simulink model "multicoptero"  (R2024b)
settings: Solver=FixedStepAuto  StartTime=0.0  StopTime=10  FixedStep=1e-3  RelTol=1e-3
undefined symbols (not defined in the file or in its folder): carga, controlador, planta
libraries: slpidlib x6
settings Model: Creator=mmaximo  LastModifiedBy=guicr
settings SolverCC: AlgebraicLoopSolver=TrustRegion
settings DebuggingCC: UnconnectedInputMsg=warning  UnconnectedOutputMsg=warning  UnconnectedLineMsg=warning
settings ModelReferenceCC: EnableRefExpFcnMdlSchedulingChecks=on
settings RTWCC: GPUComputeCapability=3.5

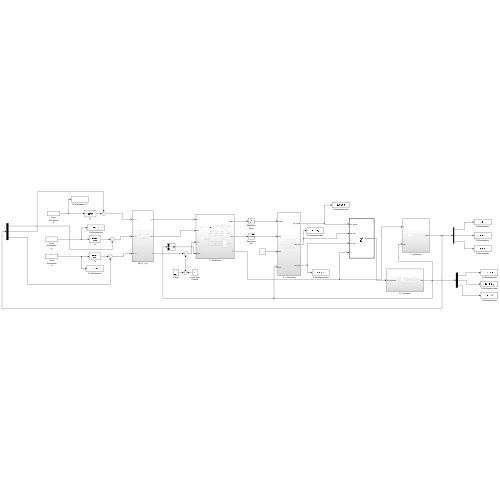
[thumbnail: Simulink's stored preview of the top-level diagram]
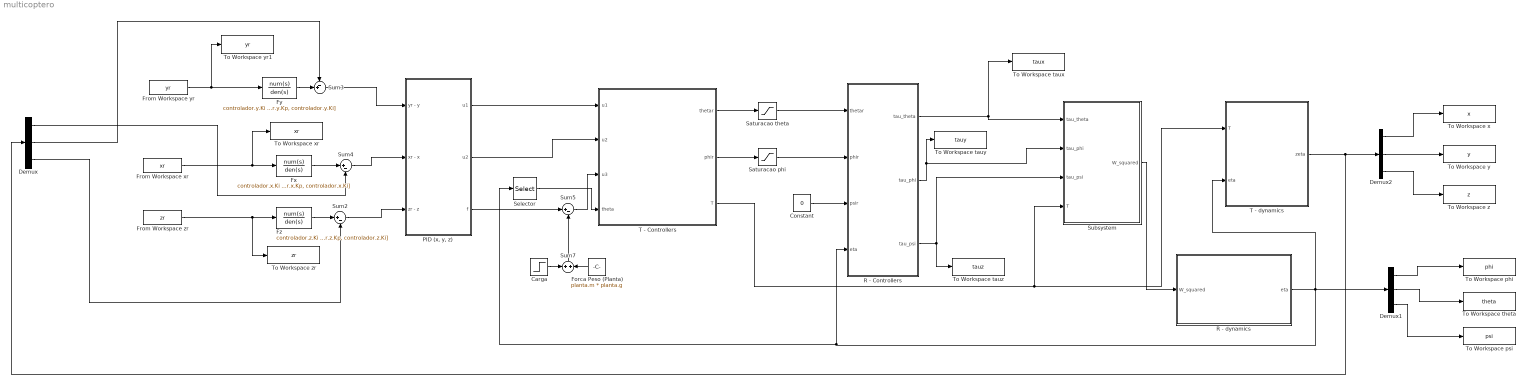
== system multicoptero ==
  Carga : Step  Time=3  After=carga * planta.g  SampleTime=0
  Constant : Constant  Value=0
  Demux : Demux  Outputs=3
  Demux1 : Demux  Outputs=3
  Demux2 : Demux  Outputs=3
  Forca Peso (Planta) : Constant  Value=planta.m * planta.g
  From Workspace xr : FromWorkspace  VariableName=xr
  From Workspace yr : FromWorkspace  VariableName=yr
  From Workspace zr : FromWorkspace  VariableName=zr
  Fx : TransferFcn  Numerator=controlador.x.Ki  Denominator=[controlador.x.Kd, controlador.x.Kp, controlador.x.Ki]
  Fy : TransferFcn  Numerator=controlador.y.Ki  Denominator=[controlador.y.Kd, controlador.y.Kp, controlador.y.Ki]
  Fz : TransferFcn  Numerator=controlador.z.Ki  Denominator=[controlador.z.Kd, controlador.z.Kp, controlador.z.Ki]
  "PID (x, y, z)" : Subsystem
  R - Controllers : Subsystem
  R - dynamics : Subsystem
  Saturacao phi : Saturate  UpperLimit=80 * pi / 180  LowerLimit=-80 * pi / 180
  Saturacao theta : Saturate  UpperLimit=80 * pi / 180  LowerLimit=-80 * pi / 180
  Selector : Selector  InputPortWidth=3  IndexOptions=Index vector (dialog)  Indices=[2]  OutputSizes=1
  Subsystem : MATLAB Function  TreatAsAtomicUnit=on
  Sum2 : Sum  Inputs=|+-
  Sum3 : Sum  Inputs=-+|
  Sum4 : Sum  Inputs=|+-
  Sum5 : Sum  Inputs=|+-
  Sum7 : Sum  Inputs=+|+
  T - Controllers : Subsystem
  T - dynamics : Subsystem
  To Workspace phi : ToWorkspace  VariableName=phi  SaveFormat=Structure With Time  SampleTime=-1
  To Workspace psi : ToWorkspace  VariableName=psi  SaveFormat=Structure With Time  SampleTime=-1
  To Workspace taux : ToWorkspace  VariableName=taux  SaveFormat=Structure With Time  SampleTime=-1
  To Workspace tauy : ToWorkspace  VariableName=tauy  SaveFormat=Structure With Time  SampleTime=-1
  To Workspace tauz : ToWorkspace  VariableName=tauz  SaveFormat=Structure With Time  SampleTime=-1
  To Workspace theta : ToWorkspace  VariableName=theta  SaveFormat=Structure With Time  SampleTime=-1
  To Workspace x : ToWorkspace  VariableName=x  SaveFormat=Structure With Time  SampleTime=-1
  To Workspace xr : ToWorkspace  VariableName=xr  SaveFormat=Structure With Time  SampleTime=-1
  To Workspace y : ToWorkspace  VariableName=y  SaveFormat=Structure With Time  SampleTime=-1
  To Workspace yr1 : ToWorkspace  VariableName=yr  SaveFormat=Structure With Time  SampleTime=-1
  To Workspace z : ToWorkspace  VariableName=z  SaveFormat=Structure With Time  SampleTime=-1
  To Workspace zr : ToWorkspace  VariableName=zr  SaveFormat=Structure With Time  SampleTime=-1
  wires:
  From Workspace yr/1 -> To Workspace yr1/1, Fy/1
  From Workspace zr/1 -> Fz/1, To Workspace zr/1
  Fz/1 -> Sum2/1
  Fx/1 -> Sum4/1
  From Workspace xr/1 -> To Workspace xr/1, Fx/1
  Fy/1 -> Sum3/2
  Sum3/1 -> "PID (x, y, z)"/1(yr - y)
  Sum4/1 -> "PID (x, y, z)"/2(xr - x)
  Sum2/1 -> "PID (x, y, z)"/3(zr - z)
  Forca Peso (Planta)/1 -> Sum7/2
  Sum7/1 -> Sum5/2
  Carga/1 -> Sum7/1
  "PID (x, y, z)"/3(f) -> Sum5/1
  "PID (x, y, z)"/1(u1) -> T - Controllers/1(u1)
  "PID (x, y, z)"/2(u2) -> T - Controllers/2(u2)
  Sum5/1 -> T - Controllers/3(u3)
  T - Controllers/1(thetar) -> Saturacao theta/1
  T - Controllers/2(phir) -> Saturacao phi/1
  Constant/1 -> R - Controllers/3(psir)
  R - Controllers/2(tau_phi) -> Subsystem/2(tau_phi), To Workspace tauy/1
  R - Controllers/1(tau_theta) -> To Workspace taux/1, Subsystem/1(tau_theta)
  R - Controllers/3(tau_psi) -> To Workspace tauz/1, Subsystem/3(tau_psi)
  Subsystem/1(W_squared) -> R - dynamics/1(W_squared)
  Demux/3 -> Sum2/2
  Demux/1 -> Sum4/2
  Demux/2 -> Sum3/1
  R - dynamics/1(eta) -> Selector/1, R - Controllers/4(eta), Demux1/1, T - dynamics/2(eta)
  T - dynamics/1(zeta) -> Demux/1, Demux2/1
  Saturacao theta/1 -> R - Controllers/1(thetar)
  Saturacao phi/1 -> R - Controllers/2(phir)
  Demux1/1 -> To Workspace phi/1
  Demux1/2 -> To Workspace theta/1
  Demux1/3 -> To Workspace psi/1
  Demux2/1 -> To Workspace x/1
  Demux2/2 -> To Workspace y/1
  Demux2/3 -> To Workspace z/1
  T - Controllers/3(T) -> T - dynamics/1(T), Subsystem/4(T)
  Selector/1 -> T - Controllers/4(theta)

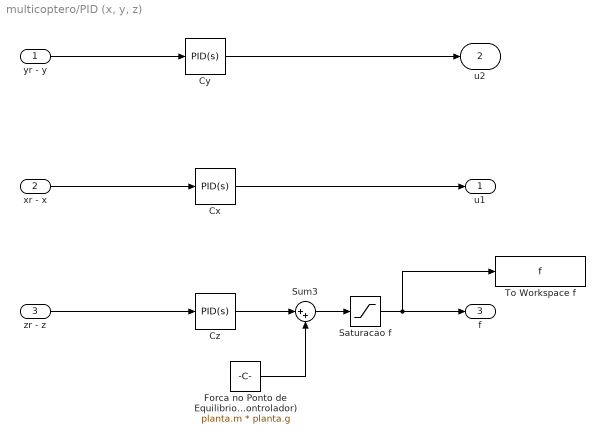
== system multicoptero/PID (x, y, z) ==
  yr - y : Inport
  xr - x : Inport  Port=2
  zr - z : Inport  Port=3
  Cx : slpidlib/PID Controller  Controller=PID  Form=Parallel  TimeDomain=Continuous-time  UseExternalTs=off  SampleTime=-1  IntegratorMethod=Forward Euler  FilterMethod=Forward Euler  ControllerParametersSource=internal  P=controlador.x.Kp  I=controlador.x.Ki  UseKiTs=off  D=controlador.x.Kd  UseExternalDerivativeSource=off  N=100  UseFilter=on  TunerSelectOption=Transfer Function Based (PID Tuner App)  InitialConditionSource=internal  InitialConditionForIntegrator=0  InitialConditionForFilter=0  DifferentiatorICPrevScaledInput=0  ExternalReset=none  TrackingMode=off  Kt=1  LimitOutput=off  SatLimitsSource=internal  UpperSaturationLimit=inf  LowerSaturationLimit=-inf  LinearizeAsGain=on  AntiWindupMode=none  Kb=1  LimitIntegrator=off  UpperIntegratorSaturationLimit=inf  LowerIntegratorSaturationLimit=-inf  POutMin=[]  POutMax=[]  IOutMin=[]  IOutMax=[]  DOutMin=[]  DOutMax=[]  NOutMin=[]  NOutMax=[]  SumOutMin=[]  SumOutMax=[]  SaturationOutMin=[]  SaturationOutMax=[]  PParamMin=[]  PParamMax=[]  IParamMin=[]  IParamMax=[]  DParamMin=[]  DParamMax=[]  NParamMin=[]  NParamMax=[]  KbParamMin=[]  KbParamMax=[]  KtParamMin=[]  KtParamMax=[]  KbOutMin=[]  KbOutMax=[]  KtOutMin=[]  KtOutMax=[]  IntegratorOutMin=[]  IntegratorOutMax=[]  FilterOutMin=[]  FilterOutMax=[]  SumI1OutMin=[]  SumI1OutMax=[]  SumI2OutMin=[]  SumI2OutMax=[]  SumI3OutMin=[]  SumI3OutMax=[]  SumI4OutMin=[]  SumI4OutMax=[]  SumDOutMin=[]  SumDOutMax=[]  DifferentiatorOutMin=[]  DifferentiatorOutMax=[]  FilterDiffOutCoefMin=[]  FilterDiffOutCoefMax=[]  ReciprocalOutMin=[]  ReciprocalOutMax=[]  SumDenOutMin=[]  SumDenOutMax=[]  SumNumOutMin=[]  SumNumOutMax=[]  DivideOutMin=[]  DivideOutMax=[]  UdiffTsProdOutMin=[]  UdiffTsProdOutMax=[]  NTsProdOutMin=[]  NTsProdOutMax=[]  UintegralTsProdOutMin=[]  UintegralTsProdOutMax=[]  UngainTsProdOutMin=[]  UngainTsProdOutMax=[]  ClampingZeroOutDataTypeStr=Inherit: Inherit via back propagation  ClampingZeroOutMin=[]  ClampingZeroOutMax=[]  FilterDenConstantOutDataTypeStr=Inherit: Inherit via back propagation  FilterDenConstantOutMin=[]  FilterDenConstantOutMax=[]  PCopyOutDataTypeStr=Inherit: Inherit via back propagation  PCopyOutMin=[]  PCopyOutMax=[]  NCopyOutDataTypeStr=Inherit: Inherit via back propagation  NCopyOutMin=[]  NCopyOutMax=[]  IntegratorContinuousStateAttributes=''  IntegratorStateMustResolveToSignalObject=off  IntegratorRTWStateStorageClass=Auto  FilterContinuousStateAttributes=''  FilterStateMustResolveToSignalObject=off  FilterRTWStateStorageClass=Auto  ParallelPVariant=InternalParameters  IdealPVariant=Disabled  IVariant=InternalParameters  DVariant=InternalParameters  IntegratorVariant=Continuous  SatVariant=Disabled  AWVariant=Passthrough  PCopyVariant=Disabled  TRVariant=Disabled  FdbkBlocksVariant=Forward  IdealPFdbkVariant=Disabled  SatFdbkVariant=Disabled  DerivativeFilterVariant=ContFilter  NVariant=InternalParameters  NCopyVariant=Disabled  FilterICVariant=InternalICsFilter  IntegratorICVariant=InternalICs  ExternalResetVariant=Disabled  TRSumVariant=Passthrough  SumFdbkVariant=Disabled  SumVariant=Sum_PID  TsampFilterVariant=InternalTs  TsampNgainVariant=Passthrough  TsampIntegralVariant=Disabled_SignalSpec  ExternalSaturationOutDataTypeStr=Inherit: Same as second input  DerivativeSourceVariant=ErrorSignal  PreIntVariant=InternalPreInt
  Cy : slpidlib/PID Controller  Controller=PID  Form=Parallel  TimeDomain=Continuous-time  UseExternalTs=off  SampleTime=-1  IntegratorMethod=Forward Euler  FilterMethod=Forward Euler  ControllerParametersSource=internal  P=controlador.y.Kp  I=controlador.y.Ki  UseKiTs=off  D=controlador.y.Kd  UseExternalDerivativeSource=off  N=100  UseFilter=on  TunerSelectOption=Transfer Function Based (PID Tuner App)  InitialConditionSource=internal  InitialConditionForIntegrator=0  InitialConditionForFilter=0  DifferentiatorICPrevScaledInput=0  ExternalReset=none  TrackingMode=off  Kt=1  LimitOutput=off  SatLimitsSource=internal  UpperSaturationLimit=inf  LowerSaturationLimit=-inf  LinearizeAsGain=on  AntiWindupMode=none  Kb=1  LimitIntegrator=off  UpperIntegratorSaturationLimit=inf  LowerIntegratorSaturationLimit=-inf  POutMin=[]  POutMax=[]  IOutMin=[]  IOutMax=[]  DOutMin=[]  DOutMax=[]  NOutMin=[]  NOutMax=[]  SumOutMin=[]  SumOutMax=[]  SaturationOutMin=[]  SaturationOutMax=[]  PParamMin=[]  PParamMax=[]  IParamMin=[]  IParamMax=[]  DParamMin=[]  DParamMax=[]  NParamMin=[]  NParamMax=[]  KbParamMin=[]  KbParamMax=[]  KtParamMin=[]  KtParamMax=[]  KbOutMin=[]  KbOutMax=[]  KtOutMin=[]  KtOutMax=[]  IntegratorOutMin=[]  IntegratorOutMax=[]  FilterOutMin=[]  FilterOutMax=[]  SumI1OutMin=[]  SumI1OutMax=[]  SumI2OutMin=[]  SumI2OutMax=[]  SumI3OutMin=[]  SumI3OutMax=[]  SumI4OutMin=[]  SumI4OutMax=[]  SumDOutMin=[]  SumDOutMax=[]  DifferentiatorOutMin=[]  DifferentiatorOutMax=[]  FilterDiffOutCoefMin=[]  FilterDiffOutCoefMax=[]  ReciprocalOutMin=[]  ReciprocalOutMax=[]  SumDenOutMin=[]  SumDenOutMax=[]  SumNumOutMin=[]  SumNumOutMax=[]  DivideOutMin=[]  DivideOutMax=[]  UdiffTsProdOutMin=[]  UdiffTsProdOutMax=[]  NTsProdOutMin=[]  NTsProdOutMax=[]  UintegralTsProdOutMin=[]  UintegralTsProdOutMax=[]  UngainTsProdOutMin=[]  UngainTsProdOutMax=[]  ClampingZeroOutDataTypeStr=Inherit: Inherit via back propagation  ClampingZeroOutMin=[]  ClampingZeroOutMax=[]  FilterDenConstantOutDataTypeStr=Inherit: Inherit via back propagation  FilterDenConstantOutMin=[]  FilterDenConstantOutMax=[]  PCopyOutDataTypeStr=Inherit: Inherit via back propagation  PCopyOutMin=[]  PCopyOutMax=[]  NCopyOutDataTypeStr=Inherit: Inherit via back propagation  NCopyOutMin=[]  NCopyOutMax=[]  IntegratorContinuousStateAttributes=''  IntegratorStateMustResolveToSignalObject=off  IntegratorRTWStateStorageClass=Auto  FilterContinuousStateAttributes=''  FilterStateMustResolveToSignalObject=off  FilterRTWStateStorageClass=Auto  ParallelPVariant=InternalParameters  IdealPVariant=Disabled  IVariant=InternalParameters  DVariant=InternalParameters  IntegratorVariant=Continuous  SatVariant=Disabled  AWVariant=Passthrough  PCopyVariant=Disabled  TRVariant=Disabled  FdbkBlocksVariant=Forward  IdealPFdbkVariant=Disabled  SatFdbkVariant=Disabled  DerivativeFilterVariant=ContFilter  NVariant=InternalParameters  NCopyVariant=Disabled  FilterICVariant=InternalICsFilter  IntegratorICVariant=InternalICs  ExternalResetVariant=Disabled  TRSumVariant=Passthrough  SumFdbkVariant=Disabled  SumVariant=Sum_PID  TsampFilterVariant=InternalTs  TsampNgainVariant=Passthrough  TsampIntegralVariant=Disabled_SignalSpec  ExternalSaturationOutDataTypeStr=Inherit: Same as second input  DerivativeSourceVariant=ErrorSignal  PreIntVariant=InternalPreInt
  Cz : slpidlib/PID Controller  Controller=PID  Form=Parallel  TimeDomain=Continuous-time  UseExternalTs=off  SampleTime=-1  IntegratorMethod=Forward Euler  FilterMethod=Forward Euler  ControllerParametersSource=internal  P=controlador.z.Kp  I=controlador.z.Ki  UseKiTs=off  D=controlador.z.Kd  UseExternalDerivativeSource=off  N=100  UseFilter=on  TunerSelectOption=Transfer Function Based (PID Tuner App)  InitialConditionSource=internal  InitialConditionForIntegrator=0  InitialConditionForFilter=0  DifferentiatorICPrevScaledInput=0  ExternalReset=none  TrackingMode=off  Kt=1  LimitOutput=off  SatLimitsSource=internal  UpperSaturationLimit=inf  LowerSaturationLimit=-inf  LinearizeAsGain=on  AntiWindupMode=none  Kb=1  LimitIntegrator=off  UpperIntegratorSaturationLimit=inf  LowerIntegratorSaturationLimit=-inf  POutMin=[]  POutMax=[]  IOutMin=[]  IOutMax=[]  DOutMin=[]  DOutMax=[]  NOutMin=[]  NOutMax=[]  SumOutMin=[]  SumOutMax=[]  SaturationOutMin=[]  SaturationOutMax=[]  PParamMin=[]  PParamMax=[]  IParamMin=[]  IParamMax=[]  DParamMin=[]  DParamMax=[]  NParamMin=[]  NParamMax=[]  KbParamMin=[]  KbParamMax=[]  KtParamMin=[]  KtParamMax=[]  KbOutMin=[]  KbOutMax=[]  KtOutMin=[]  KtOutMax=[]  IntegratorOutMin=[]  IntegratorOutMax=[]  FilterOutMin=[]  FilterOutMax=[]  SumI1OutMin=[]  SumI1OutMax=[]  SumI2OutMin=[]  SumI2OutMax=[]  SumI3OutMin=[]  SumI3OutMax=[]  SumI4OutMin=[]  SumI4OutMax=[]  SumDOutMin=[]  SumDOutMax=[]  DifferentiatorOutMin=[]  DifferentiatorOutMax=[]  FilterDiffOutCoefMin=[]  FilterDiffOutCoefMax=[]  ReciprocalOutMin=[]  ReciprocalOutMax=[]  SumDenOutMin=[]  SumDenOutMax=[]  SumNumOutMin=[]  SumNumOutMax=[]  DivideOutMin=[]  DivideOutMax=[]  UdiffTsProdOutMin=[]  UdiffTsProdOutMax=[]  NTsProdOutMin=[]  NTsProdOutMax=[]  UintegralTsProdOutMin=[]  UintegralTsProdOutMax=[]  UngainTsProdOutMin=[]  UngainTsProdOutMax=[]  ClampingZeroOutDataTypeStr=Inherit: Inherit via back propagation  ClampingZeroOutMin=[]  ClampingZeroOutMax=[]  FilterDenConstantOutDataTypeStr=Inherit: Inherit via back propagation  FilterDenConstantOutMin=[]  FilterDenConstantOutMax=[]  PCopyOutDataTypeStr=Inherit: Inherit via back propagation  PCopyOutMin=[]  PCopyOutMax=[]  NCopyOutDataTypeStr=Inherit: Inherit via back propagation  NCopyOutMin=[]  NCopyOutMax=[]  IntegratorContinuousStateAttributes=''  IntegratorStateMustResolveToSignalObject=off  IntegratorRTWStateStorageClass=Auto  FilterContinuousStateAttributes=''  FilterStateMustResolveToSignalObject=off  FilterRTWStateStorageClass=Auto  ParallelPVariant=InternalParameters  IdealPVariant=Disabled  IVariant=InternalParameters  DVariant=InternalParameters  IntegratorVariant=Continuous  SatVariant=Disabled  AWVariant=Passthrough  PCopyVariant=Disabled  TRVariant=Disabled  FdbkBlocksVariant=Forward  IdealPFdbkVariant=Disabled  SatFdbkVariant=Disabled  DerivativeFilterVariant=ContFilter  NVariant=InternalParameters  NCopyVariant=Disabled  FilterICVariant=InternalICsFilter  IntegratorICVariant=InternalICs  ExternalResetVariant=Disabled  TRSumVariant=Passthrough  SumFdbkVariant=Disabled  SumVariant=Sum_PID  TsampFilterVariant=InternalTs  TsampNgainVariant=Passthrough  TsampIntegralVariant=Disabled_SignalSpec  ExternalSaturationOutDataTypeStr=Inherit: Same as second input  DerivativeSourceVariant=ErrorSignal  PreIntVariant=InternalPreInt
  Forca no Ponto de Equilibrio f0 (Controlador) : Constant  Value=planta.m * planta.g
  Saturacao f : Saturate  UpperLimit=1.8 * planta.m * planta.g  LowerLimit=0.2 * planta.m * planta.g
  Sum3 : Sum  Inputs=|++
  To Workspace f : ToWorkspace  VariableName=f  SaveFormat=Structure With Time  SampleTime=-1
  u1 : Outport
  u2 : Outport  Port=2
  f : Outport  Port=3
  wires:
  Forca no Ponto de Equilibrio f0 (Controlador)/1 -> Sum3/2
  Cx/1 -> u1/1
  xr - x/1 -> Cx/1
  Saturacao f/1 -> To Workspace f/1, f/1
  Cz/1 -> Sum3/1
  Cy/1 -> u2/1
  Sum3/1 -> Saturacao f/1
  yr - y/1 -> Cy/1
  zr - z/1 -> Cz/1

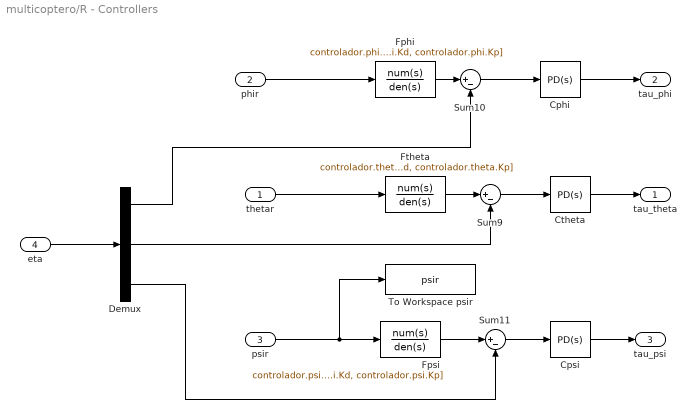
== system multicoptero/R - Controllers ==
  thetar : Inport
  phir : Inport  Port=2
  psir : Inport  Port=3
  eta : Inport  Port=4
  Cphi : slpidlib/PID Controller  Controller=PD  Form=Parallel  TimeDomain=Continuous-time  UseExternalTs=off  SampleTime=-1  IntegratorMethod=Forward Euler  FilterMethod=Forward Euler  ControllerParametersSource=internal  P=controlador.phi.Kp  I=controlador.phi.Ki  UseKiTs=off  D=controlador.phi.Kd  UseExternalDerivativeSource=off  N=100  UseFilter=on  TunerSelectOption=Transfer Function Based (PID Tuner App)  InitialConditionSource=internal  InitialConditionForIntegrator=0  InitialConditionForFilter=0  DifferentiatorICPrevScaledInput=0  ExternalReset=none  TrackingMode=off  Kt=1  LimitOutput=off  SatLimitsSource=internal  UpperSaturationLimit=inf  LowerSaturationLimit=-inf  LinearizeAsGain=on  AntiWindupMode=none  Kb=1  LimitIntegrator=off  UpperIntegratorSaturationLimit=inf  LowerIntegratorSaturationLimit=-inf  POutMin=[]  POutMax=[]  IOutMin=[]  IOutMax=[]  DOutMin=[]  DOutMax=[]  NOutMin=[]  NOutMax=[]  SumOutMin=[]  SumOutMax=[]  SaturationOutMin=[]  SaturationOutMax=[]  PParamMin=[]  PParamMax=[]  IParamMin=[]  IParamMax=[]  DParamMin=[]  DParamMax=[]  NParamMin=[]  NParamMax=[]  KbParamMin=[]  KbParamMax=[]  KtParamMin=[]  KtParamMax=[]  KbOutMin=[]  KbOutMax=[]  KtOutMin=[]  KtOutMax=[]  IntegratorOutMin=[]  IntegratorOutMax=[]  FilterOutMin=[]  FilterOutMax=[]  SumI1OutMin=[]  SumI1OutMax=[]  SumI2OutMin=[]  SumI2OutMax=[]  SumI3OutMin=[]  SumI3OutMax=[]  SumI4OutMin=[]  SumI4OutMax=[]  SumDOutMin=[]  SumDOutMax=[]  DifferentiatorOutMin=[]  DifferentiatorOutMax=[]  FilterDiffOutCoefMin=[]  FilterDiffOutCoefMax=[]  ReciprocalOutMin=[]  ReciprocalOutMax=[]  SumDenOutMin=[]  SumDenOutMax=[]  SumNumOutMin=[]  SumNumOutMax=[]  DivideOutMin=[]  DivideOutMax=[]  UdiffTsProdOutMin=[]  UdiffTsProdOutMax=[]  NTsProdOutMin=[]  NTsProdOutMax=[]  UintegralTsProdOutMin=[]  UintegralTsProdOutMax=[]  UngainTsProdOutMin=[]  UngainTsProdOutMax=[]  ClampingZeroOutDataTypeStr=Inherit: Inherit via back propagation  ClampingZeroOutMin=[]  ClampingZeroOutMax=[]  FilterDenConstantOutDataTypeStr=Inherit: Inherit via back propagation  FilterDenConstantOutMin=[]  FilterDenConstantOutMax=[]  PCopyOutDataTypeStr=Inherit: Inherit via back propagation  PCopyOutMin=[]  PCopyOutMax=[]  NCopyOutDataTypeStr=Inherit: Inherit via back propagation  NCopyOutMin=[]  NCopyOutMax=[]  IntegratorContinuousStateAttributes=''  IntegratorStateMustResolveToSignalObject=off  IntegratorRTWStateStorageClass=Auto  FilterContinuousStateAttributes=''  FilterStateMustResolveToSignalObject=off  FilterRTWStateStorageClass=Auto  ParallelPVariant=InternalParameters  IdealPVariant=Disabled  IVariant=Disabled  DVariant=InternalParameters  IntegratorVariant=Disabled  SatVariant=Disabled  AWVariant=Disabled  PCopyVariant=Disabled  TRVariant=Disabled  FdbkBlocksVariant=Forward  IdealPFdbkVariant=Disabled  SatFdbkVariant=Disabled  DerivativeFilterVariant=ContFilter  NVariant=InternalParameters  NCopyVariant=Disabled  FilterICVariant=InternalICsFilter  IntegratorICVariant=Disabled  ExternalResetVariant=Disabled  TRSumVariant=Passthrough  SumFdbkVariant=Disabled  SumVariant=Sum_PD  TsampFilterVariant=InternalTs  TsampNgainVariant=Passthrough  TsampIntegralVariant=Disabled_SignalSpec  ExternalSaturationOutDataTypeStr=Inherit: Same as second input  DerivativeSourceVariant=ErrorSignal  PreIntVariant=InternalPreInt
  Cpsi : slpidlib/PID Controller  Controller=PD  Form=Parallel  TimeDomain=Continuous-time  UseExternalTs=off  SampleTime=-1  IntegratorMethod=Forward Euler  FilterMethod=Forward Euler  ControllerParametersSource=internal  P=controlador.psi.Kp  I=controlador.psi.Ki  UseKiTs=off  D=controlador.psi.Kd  UseExternalDerivativeSource=off  N=100  UseFilter=on  TunerSelectOption=Transfer Function Based (PID Tuner App)  InitialConditionSource=internal  InitialConditionForIntegrator=0  InitialConditionForFilter=0  DifferentiatorICPrevScaledInput=0  ExternalReset=none  TrackingMode=off  Kt=1  LimitOutput=off  SatLimitsSource=internal  UpperSaturationLimit=inf  LowerSaturationLimit=-inf  LinearizeAsGain=on  AntiWindupMode=none  Kb=1  LimitIntegrator=off  UpperIntegratorSaturationLimit=inf  LowerIntegratorSaturationLimit=-inf  POutMin=[]  POutMax=[]  IOutMin=[]  IOutMax=[]  DOutMin=[]  DOutMax=[]  NOutMin=[]  NOutMax=[]  SumOutMin=[]  SumOutMax=[]  SaturationOutMin=[]  SaturationOutMax=[]  PParamMin=[]  PParamMax=[]  IParamMin=[]  IParamMax=[]  DParamMin=[]  DParamMax=[]  NParamMin=[]  NParamMax=[]  KbParamMin=[]  KbParamMax=[]  KtParamMin=[]  KtParamMax=[]  KbOutMin=[]  KbOutMax=[]  KtOutMin=[]  KtOutMax=[]  IntegratorOutMin=[]  IntegratorOutMax=[]  FilterOutMin=[]  FilterOutMax=[]  SumI1OutMin=[]  SumI1OutMax=[]  SumI2OutMin=[]  SumI2OutMax=[]  SumI3OutMin=[]  SumI3OutMax=[]  SumI4OutMin=[]  SumI4OutMax=[]  SumDOutMin=[]  SumDOutMax=[]  DifferentiatorOutMin=[]  DifferentiatorOutMax=[]  FilterDiffOutCoefMin=[]  FilterDiffOutCoefMax=[]  ReciprocalOutMin=[]  ReciprocalOutMax=[]  SumDenOutMin=[]  SumDenOutMax=[]  SumNumOutMin=[]  SumNumOutMax=[]  DivideOutMin=[]  DivideOutMax=[]  UdiffTsProdOutMin=[]  UdiffTsProdOutMax=[]  NTsProdOutMin=[]  NTsProdOutMax=[]  UintegralTsProdOutMin=[]  UintegralTsProdOutMax=[]  UngainTsProdOutMin=[]  UngainTsProdOutMax=[]  ClampingZeroOutDataTypeStr=Inherit: Inherit via back propagation  ClampingZeroOutMin=[]  ClampingZeroOutMax=[]  FilterDenConstantOutDataTypeStr=Inherit: Inherit via back propagation  FilterDenConstantOutMin=[]  FilterDenConstantOutMax=[]  PCopyOutDataTypeStr=Inherit: Inherit via back propagation  PCopyOutMin=[]  PCopyOutMax=[]  NCopyOutDataTypeStr=Inherit: Inherit via back propagation  NCopyOutMin=[]  NCopyOutMax=[]  IntegratorContinuousStateAttributes=''  IntegratorStateMustResolveToSignalObject=off  IntegratorRTWStateStorageClass=Auto  FilterContinuousStateAttributes=''  FilterStateMustResolveToSignalObject=off  FilterRTWStateStorageClass=Auto  ParallelPVariant=InternalParameters  IdealPVariant=Disabled  IVariant=Disabled  DVariant=InternalParameters  IntegratorVariant=Disabled  SatVariant=Disabled  AWVariant=Disabled  PCopyVariant=Disabled  TRVariant=Disabled  FdbkBlocksVariant=Forward  IdealPFdbkVariant=Disabled  SatFdbkVariant=Disabled  DerivativeFilterVariant=ContFilter  NVariant=InternalParameters  NCopyVariant=Disabled  FilterICVariant=InternalICsFilter  IntegratorICVariant=Disabled  ExternalResetVariant=Disabled  TRSumVariant=Passthrough  SumFdbkVariant=Disabled  SumVariant=Sum_PD  TsampFilterVariant=InternalTs  TsampNgainVariant=Passthrough  TsampIntegralVariant=Disabled_SignalSpec  ExternalSaturationOutDataTypeStr=Inherit: Same as second input  DerivativeSourceVariant=ErrorSignal  PreIntVariant=InternalPreInt
  Ctheta : slpidlib/PID Controller  Controller=PD  Form=Parallel  TimeDomain=Continuous-time  UseExternalTs=off  SampleTime=-1  IntegratorMethod=Forward Euler  FilterMethod=Forward Euler  ControllerParametersSource=internal  P=controlador.theta.Kp  I=controlador.theta.Ki  UseKiTs=off  D=controlador.theta.Kd  UseExternalDerivativeSource=off  N=100  UseFilter=on  TunerSelectOption=Transfer Function Based (PID Tuner App)  InitialConditionSource=internal  InitialConditionForIntegrator=0  InitialConditionForFilter=0  DifferentiatorICPrevScaledInput=0  ExternalReset=none  TrackingMode=off  Kt=1  LimitOutput=off  SatLimitsSource=internal  UpperSaturationLimit=inf  LowerSaturationLimit=-inf  LinearizeAsGain=on  AntiWindupMode=none  Kb=1  LimitIntegrator=off  UpperIntegratorSaturationLimit=inf  LowerIntegratorSaturationLimit=-inf  POutMin=[]  POutMax=[]  IOutMin=[]  IOutMax=[]  DOutMin=[]  DOutMax=[]  NOutMin=[]  NOutMax=[]  SumOutMin=[]  SumOutMax=[]  SaturationOutMin=[]  SaturationOutMax=[]  PParamMin=[]  PParamMax=[]  IParamMin=[]  IParamMax=[]  DParamMin=[]  DParamMax=[]  NParamMin=[]  NParamMax=[]  KbParamMin=[]  KbParamMax=[]  KtParamMin=[]  KtParamMax=[]  KbOutMin=[]  KbOutMax=[]  KtOutMin=[]  KtOutMax=[]  IntegratorOutMin=[]  IntegratorOutMax=[]  FilterOutMin=[]  FilterOutMax=[]  SumI1OutMin=[]  SumI1OutMax=[]  SumI2OutMin=[]  SumI2OutMax=[]  SumI3OutMin=[]  SumI3OutMax=[]  SumI4OutMin=[]  SumI4OutMax=[]  SumDOutMin=[]  SumDOutMax=[]  DifferentiatorOutMin=[]  DifferentiatorOutMax=[]  FilterDiffOutCoefMin=[]  FilterDiffOutCoefMax=[]  ReciprocalOutMin=[]  ReciprocalOutMax=[]  SumDenOutMin=[]  SumDenOutMax=[]  SumNumOutMin=[]  SumNumOutMax=[]  DivideOutMin=[]  DivideOutMax=[]  UdiffTsProdOutMin=[]  UdiffTsProdOutMax=[]  NTsProdOutMin=[]  NTsProdOutMax=[]  UintegralTsProdOutMin=[]  UintegralTsProdOutMax=[]  UngainTsProdOutMin=[]  UngainTsProdOutMax=[]  ClampingZeroOutDataTypeStr=Inherit: Inherit via back propagation  ClampingZeroOutMin=[]  ClampingZeroOutMax=[]  FilterDenConstantOutDataTypeStr=Inherit: Inherit via back propagation  FilterDenConstantOutMin=[]  FilterDenConstantOutMax=[]  PCopyOutDataTypeStr=Inherit: Inherit via back propagation  PCopyOutMin=[]  PCopyOutMax=[]  NCopyOutDataTypeStr=Inherit: Inherit via back propagation  NCopyOutMin=[]  NCopyOutMax=[]  IntegratorContinuousStateAttributes=''  IntegratorStateMustResolveToSignalObject=off  IntegratorRTWStateStorageClass=Auto  FilterContinuousStateAttributes=''  FilterStateMustResolveToSignalObject=off  FilterRTWStateStorageClass=Auto  ParallelPVariant=InternalParameters  IdealPVariant=Disabled  IVariant=Disabled  DVariant=InternalParameters  IntegratorVariant=Disabled  SatVariant=Disabled  AWVariant=Disabled  PCopyVariant=Disabled  TRVariant=Disabled  FdbkBlocksVariant=Forward  IdealPFdbkVariant=Disabled  SatFdbkVariant=Disabled  DerivativeFilterVariant=ContFilter  NVariant=InternalParameters  NCopyVariant=Disabled  FilterICVariant=InternalICsFilter  IntegratorICVariant=Disabled  ExternalResetVariant=Disabled  TRSumVariant=Passthrough  SumFdbkVariant=Disabled  SumVariant=Sum_PD  TsampFilterVariant=InternalTs  TsampNgainVariant=Passthrough  TsampIntegralVariant=Disabled_SignalSpec  ExternalSaturationOutDataTypeStr=Inherit: Same as second input  DerivativeSourceVariant=ErrorSignal  PreIntVariant=InternalPreInt
  Demux : Demux  Outputs=3
  Fphi : TransferFcn  Numerator=controlador.phi.Kp  Denominator=[controlador.phi.Kd, controlador.phi.Kp]
  Fpsi : TransferFcn  Numerator=controlador.psi.Kp  Denominator=[controlador.psi.Kd, controlador.psi.Kp]
  Ftheta : TransferFcn  Numerator=controlador.theta.Kp  Denominator=[controlador.theta.Kd, controlador.theta.Kp]
  Sum10 : Sum  Inputs=|+-
  Sum11 : Sum  Inputs=|+-
  Sum9 : Sum  Inputs=|+-
  To Workspace psir : ToWorkspace  VariableName=psir  SaveFormat=Structure With Time  SampleTime=-1
  tau_theta : Outport
  tau_phi : Outport  Port=2
  tau_psi : Outport  Port=3
  wires:
  psir/1 -> To Workspace psir/1, Fpsi/1
  Sum9/1 -> Ctheta/1
  Sum10/1 -> Cphi/1
  Fpsi/1 -> Sum11/1
  Fphi/1 -> Sum10/1
  Ftheta/1 -> Sum9/1
  Sum11/1 -> Cpsi/1
  Demux/1 -> Sum10/2
  Demux/2 -> Sum9/2
  Demux/3 -> Sum11/2
  thetar/1 -> Ftheta/1
  phir/1 -> Fphi/1
  eta/1 -> Demux/1
  Cpsi/1 -> tau_psi/1
  Ctheta/1 -> tau_theta/1
  Cphi/1 -> tau_phi/1

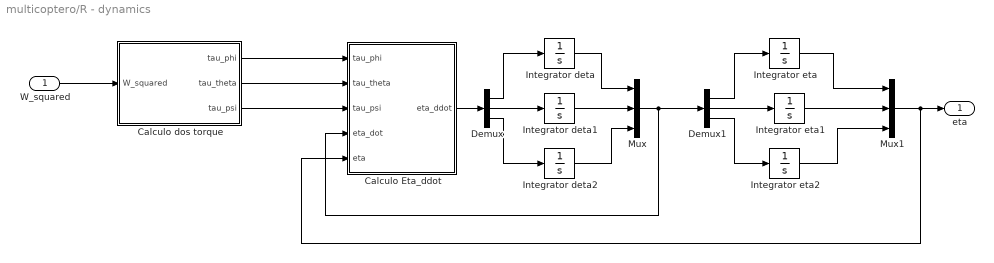
== system multicoptero/R - dynamics ==
  W_squared : Inport
  Calculo Eta_ddot : MATLAB Function  TreatAsAtomicUnit=on
  Calculo dos torque : MATLAB Function  TreatAsAtomicUnit=on
  Demux : Demux  Outputs=3
  Demux1 : Demux  Outputs=3
  Integrator deta : Integrator
  Integrator deta1 : Integrator
  Integrator deta2 : Integrator
  Integrator eta : Integrator
  Integrator eta1 : Integrator
  Integrator eta2 : Integrator
  Mux : Mux  Inputs=3
  Mux1 : Mux  Inputs=3
  eta : Outport
  wires:
  Calculo dos torque/2(tau_theta) -> Calculo Eta_ddot/2(tau_theta)
  Calculo dos torque/3(tau_psi) -> Calculo Eta_ddot/3(tau_psi)
  W_squared/1 -> Calculo dos torque/1(W_squared)
  Calculo dos torque/1(tau_phi) -> Calculo Eta_ddot/1(tau_phi)
  Demux/2 -> Integrator deta1/1
  Demux/1 -> Integrator deta/1
  Demux/3 -> Integrator deta2/1
  Calculo Eta_ddot/1(eta_ddot) -> Demux/1
  Integrator deta2/1 -> Mux/3
  Integrator deta/1 -> Mux/1
  Integrator deta1/1 -> Mux/2
  Demux1/3 -> Integrator eta2/1
  Demux1/1 -> Integrator eta/1
  Mux/1 -> Demux1/1, Calculo Eta_ddot/4(eta_dot)
  Demux1/2 -> Integrator eta1/1
  Mux1/1 -> Calculo Eta_ddot/5(eta), eta/1
  Integrator eta1/1 -> Mux1/2
  Integrator eta2/1 -> Mux1/3
  Integrator eta/1 -> Mux1/1

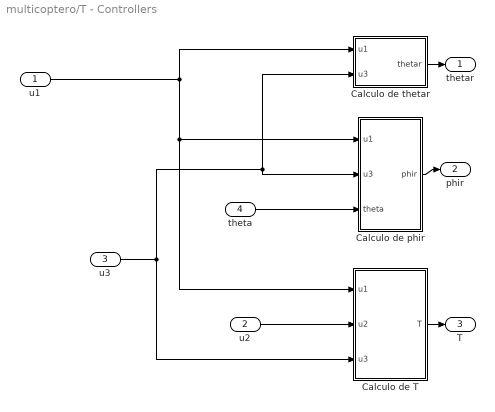
== system multicoptero/T - Controllers ==
  u1 : Inport
  u2 : Inport  Port=2
  u3 : Inport  Port=3
  theta : Inport  Port=4
  Calculo de T : MATLAB Function  TreatAsAtomicUnit=on
  Calculo de phir : MATLAB Function  TreatAsAtomicUnit=on
  Calculo de thetar : MATLAB Function  TreatAsAtomicUnit=on
  thetar : Outport
  phir : Outport  Port=2
  T : Outport  Port=3
  wires:
  u2/1 -> Calculo de T/2(u2)
  u3/1 -> Calculo de T/3(u3), Calculo de phir/2(u3), Calculo de thetar/2(u3)
  u1/1 -> Calculo de thetar/1(u1), Calculo de T/1(u1), Calculo de phir/1(u1)
  Calculo de T/1(T) -> T/1
  Calculo de phir/1(phir) -> phir/1
  Calculo de thetar/1(thetar) -> thetar/1
  theta/1 -> Calculo de phir/3(theta)

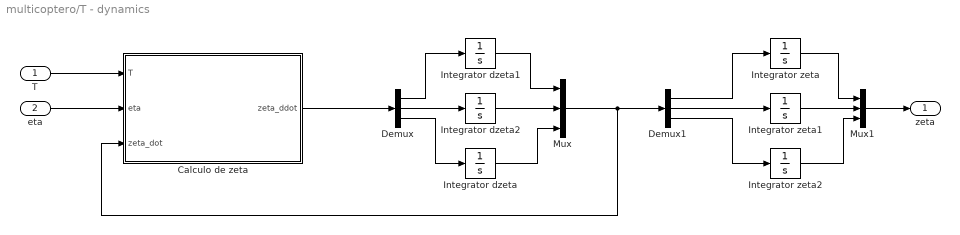
== system multicoptero/T - dynamics ==
  T : Inport
  eta : Inport  Port=2
  Calculo de zeta : MATLAB Function  TreatAsAtomicUnit=on
  Demux : Demux  Outputs=3
  Demux1 : Demux  Outputs=3
  Integrator dzeta : Integrator
  Integrator dzeta1 : Integrator
  Integrator dzeta2 : Integrator
  Integrator zeta : Integrator
  Integrator zeta1 : Integrator
  Integrator zeta2 : Integrator
  Mux : Mux  Inputs=3
  Mux1 : Mux  Inputs=3
  zeta : Outport
  wires:
  T/1 -> Calculo de zeta/1(T)
  eta/1 -> Calculo de zeta/2(eta)
  Calculo de zeta/1(zeta_ddot) -> Demux/1
  Demux/1 -> Integrator dzeta1/1
  Demux/2 -> Integrator dzeta2/1
  Demux/3 -> Integrator dzeta/1
  Integrator dzeta1/1 -> Mux/1
  Integrator dzeta2/1 -> Mux/2
  Integrator dzeta/1 -> Mux/3
  Mux/1 -> Demux1/1, Calculo de zeta/3(zeta_dot)
  Demux1/1 -> Integrator zeta/1
  Demux1/2 -> Integrator zeta1/1
  Demux1/3 -> Integrator zeta2/1
  Integrator zeta/1 -> Mux1/1
  Integrator zeta1/1 -> Mux1/2
  Integrator zeta2/1 -> Mux1/3
  Mux1/1 -> zeta/1

== matlab function multicoptero/T - Controllers/Calculo de thetar ==
  data: u1 input; thetar output; u3 input
function thetar = fcn(u1, u3)
    thetar = atan2(u1, u3);
end

== matlab function multicoptero/T - Controllers/Calculo de T ==
  data: u1 input; T output; u2 input; u3 input
function T = fcn(u1, u2, u3)
    T = sqrt(u1^2 + u2^2 + u3^2);
end

== matlab function multicoptero/T - Controllers/Calculo de phir ==
  data: u1 input; phir output; u3 input; theta input
function phir = fcn(u1, u3, theta)
    phir = atan2(-u1 * cos(theta), u3);
end

== matlab function multicoptero/Subsystem ==
  data: tau_theta input; tau_phi input; tau_psi input; T input; W_squared output
function W_squared = fcn(tau_theta, tau_phi, tau_psi, T)
W_squared = zeros(4,1); 
planta = struct( ...
    'm', 0.468, ...
    'J', 0.004856, ...
    'Jz', 0.008801, ...
    'l', 0.225, ...
    'g', 9.81, ...
    'k', 2.98e-6, ...
    'b', 1.14e-7, ...
    'Ax', 0, ...
    'Ay', 0, ...
    'Az', 0);
w1_squared = (T/(4*planta.k)) - (tau_theta/(2*planta.k*planta.l)) - (tau_psi/(4*planta.b));
w2_squared = (T/(4*planta.k)) - (tau_phi/(2*planta.k*planta.l)) + (tau_psi/(4*planta.b));
w3_squared = (T/(4*planta.k)) + (tau_theta/(2*planta.k*planta.l)) - (tau_psi/(4*planta.b));
w4_squared = (T/(4*planta.k)) + (tau_phi/(2*planta.k*planta.l)) + (tau_psi/(4*planta.b));

W_squared(1) = w1_squared;
W_squared(2) = w2_squared;
W_squared(3) = w3_squared;
W_squared(4) = w4_squared;

end

== matlab function multicoptero/T - dynamics/Calculo de zeta ==
  data: T input; zeta_ddot output; eta input; zeta_dot input
function zeta_ddot = fcn(T, eta, zeta_dot)
zeta_ddot = zeros(3,1); 
planta = struct( ...
    'm', 0.468, ...
    'J', 0.004856, ...
    'Jz', 0.008801, ...
    'l', 0.225, ...
    'g', 9.81, ...
    'k', 2.98e-6, ...
    'b', 1.14e-7, ...
    'Ax', 0, ...
    'Ay', 0, ...
    'Az', 0);

x_dot = zeta_dot(1);
y_dot = zeta_dot(2);
z_dot = zeta_dot(3);

phi = eta(1);
theta = eta(2);
psi = eta(3);

z_ddot = (T/planta.m) * (cos(phi) * cos(theta)) - planta.g - (planta.Az/planta.m) * z_dot;

x_ddot = (T/planta.m) * (sin(phi) * sin(psi) + cos(phi) * sin(theta) * cos(psi)) ...
         - (planta.Ax/planta.m) * x_dot;

y_ddot = (T/planta.m) * (-sin(phi) * cos(psi) + cos(phi) * sin(theta) * sin(psi)) ...
         - (planta.Ay/planta.m) * y_dot;


zeta_ddot(1) = x_ddot;
zeta_ddot(2) = y_ddot;
zeta_ddot(3) = z_ddot;
end

== matlab function multicoptero/R - dynamics/Calculo dos torque ==
  data: W_squared input; tau_phi output; tau_theta output; tau_psi output
function [tau_phi, tau_theta, tau_psi] = fcn(W_squared)
w1_squared = W_squared(1);
w2_squared = W_squared(2);
w3_squared = W_squared(3);
w4_squared = W_squared(4);
planta = struct( ...
    'm', 0.468, ...
    'J', 0.004856, ...
    'Jz', 0.008801, ...
    'l', 0.225, ...
    'g', 9.81, ...
    'k', 2.98e-6, ...
    'b', 1.14e-7, ...
    'Ax', 0, ...
    'Ay', 0, ...
    'Az', 0);

tau_phi = planta.l * planta.k * (-w2_squared + w4_squared);
tau_theta = planta.l * planta.k * (-w1_squared + w3_squared);
tau_psi = planta.b * (-w1_squared + w2_squared - w3_squared + w4_squared);

end

== matlab function multicoptero/R - dynamics/Calculo Eta_ddot ==
  data: tau_phi input; eta_ddot output; tau_theta input; tau_psi input; eta_dot input; eta input
function eta_ddot = fcn(tau_phi, tau_theta, tau_psi, eta_dot, eta)

phi_dot = eta_dot(1);
theta_dot = eta_dot(2);
psi_dot = eta_dot(3);
phi = eta(1);
theta = eta(2);
eta_ddot = zeros(3,1);  % ou [phi_ddot; theta_ddot; psi_ddot]

planta = struct( ...
    'm', 0.468, ...
    'J', 0.004856, ...
    'Jz', 0.008801, ...
    'l', 0.225, ...
    'g', 9.81, ...
    'k', 2.98e-6, ...
    'b', 1.14e-7, ...
    'Ax', 0, ...
    'Ay', 0, ...
    'Az', 0);

J = zeros(3,3);
C = zeros(3,3);

J(1,1) = planta.J;
J(1,2) = 0;
J(1,3) = -planta.J * sin(theta);

J(2,1) = 0;
J(2,2) = planta.J * (cos(phi))^2 + planta.Jz * (sin(phi))^2;
J(2,3) = (planta.J - planta.Jz) * cos(phi) * sin(phi) * cos(theta);

J(3,1) = -planta.J * sin(theta);
J(3,2) = (planta.J - planta.Jz) * cos(phi) * sin(phi) * cos(theta);
J(3,3) = planta.J * (sin(theta))^2 + planta.J * (sin(phi))^2 * (cos(theta))^2 + planta.Jz * (cos(phi))^2 * (cos(theta))^2;

C(1,2) = (planta.J - planta.Jz)*(theta_dot*cos(phi)*sin(phi) + psi_dot*(sin(phi))^2 * cos(theta)) + ...
         (planta.Jz - planta.J)*psi_dot*(cos(phi))^2 * cos(theta) - planta.J*psi_dot*cos(theta);

C(1,3) = (planta.Jz - planta.J)*psi_dot*cos(phi)*sin(phi)*(cos(theta))^2;

C(2,1) = (planta.Jz - planta.J)*(theta_dot*cos(phi)*sin(phi) + psi_dot*sin(phi)*cos(phi)) + ...
         (planta.J - planta.Jz)*psi_dot*(cos(phi))^2 * cos(theta) + planta.J*psi_dot*cos(theta);

C(2,2) = (planta.Jz - planta.J)*phi_dot*cos(phi)*sin(phi);

C(2,3) = -planta.J*psi_dot*sin(theta)*cos(theta) + planta.J*psi_dot*(sin(phi))^2 * sin(theta)*cos(theta) + ...
          planta.Jz*psi_dot*(cos(phi))^2 * sin(theta)*cos(theta);

C(3,1) = (planta.J - planta.Jz)*psi_dot*(cos(theta))^2 * sin(phi)*cos(phi) - planta.J*theta_dot*cos(theta);

C(3,2) = (planta.Jz - planta.J)*(theta_dot*cos(phi)*sin(phi) + phi_dot*(sin(phi))^2 * cos(theta)) + ...
         (planta.J - planta.Jz)*phi_dot*(cos(phi))^2 * cos(theta) - ...
         planta.J*psi_dot*(sin(phi))^2 * sin(theta)*cos(theta) - ...
         planta.Jz*psi_dot*(cos(phi))^2 * sin(theta)*cos(theta);

C(3,3) = (planta.Jz - planta.J)*phi_dot*cos(phi)*sin(phi)*(cos(theta))^2 - ...
         planta.J*theta_dot*(sin(phi))^2 * cos(theta)*sin(theta) + ...
         planta.Jz*theta_dot*(cos(phi))^2 * sin(theta);

if cond(J) > 1e6
    warning('J está mal condicionada! cond(J) = %.2e', cond(J));
end


% Vetor B (torques externos)
B = [tau_phi; tau_theta; tau_psi];

eta_ddot = J \ (B - C * eta_dot);


end
